simulink model "SimscapeCrane_StepInput"  (R2015a)
settings: Solver=ode15s  StartTime=0.0  StopTime=T  RelTol=1e-3
values from neighbouring files (symbols this model uses):
  filter_denominator = cell2mat(disc_filter.den)    [test.m]
  filter_numerator = cell2mat(disc_filter.num)    [test.m]
  m = 0.47    [Params_Simscape.mat]
  MR = 1.71    [Params_Simscape.mat]
  Ts_hw = 0.01    [test.m]
  TxBreak = 0    [Params_Simscape.mat]
  TxCoulomb = 3.7489    [Params_Simscape.mat]
  TxVisc = 58.085    [Params_Simscape.mat]
  TyBreak = 0    [Params_Simscape.mat]
  TyCoulomb = 2.674    [Params_Simscape.mat]
  TzBreak = 0    [Params_Simscape.mat]
  TzCoulomb = 6.1    [Params_Simscape.mat]
  xRange = [0 0.52]    [Params_Simscape.mat]
  xZero = 0.3    [Params_Simscape.mat]
  yRange = [0 0.62]    [Params_Simscape.mat]
  yZero = 0.3    [Params_Simscape.mat]
  zRange = [0.17 0.8]    [Params_Simscape.mat]
  zZero = 0.47    [Params_Simscape.mat]
undefined symbols (not defined in the file or in its folder): Ts, X, x_init, Y, Z
undefined symbols (not defined in the file): M, TorqueMultX, TorqueMultY, TorqueMultZ, TxTrans, TyTrans, TyVisc, TzTrans, TzVisc
libraries: sm_lib x146, fl_lib x62, nesl_utility x24, elec_lib x9, simulink x9, sm_double_wishbone_suspension_lib x4, aerolibtransform2 x1
(part 1 of 15)
settings Model: Creator=jsustare  LastModifiedBy=bkhusain
settings SolverCC: MaxConsecutiveMinStep=10  AutoInsertRateTranBlk=on  InsertRTBMode=Never (minimum delay)
settings DataIOCC: LimitDataPoints=off  SaveFormat=StructureWithTime
settings HardwareCC: ProdBitPerPointer=64  ProdLargestAtomicFloat=Float  ProdIntDivRoundTo=Zero  ProdEndianess=LittleEndian  ProdHWDeviceType=Specified
settings SFSimCC: SimUserIncludeDirs=../../src
settings SFSimCC: SimUserSources=|
  | user_block.c
  | user_bounds.c
  | user_gradient.c
  | user_hessians.c
  | user_jacobians.c
  | user_residual.c
  | user_mv_mult_prescaled.c
  | user_prescaler.c
  | user_rec_sol.c
  | user_minres.c
  | user_lanczos.c
  | user_nlp_solver.c
  | soc_simulink_wrapper.c
settings GRTTargetCC: GeneratePreprocessorConditionals=Use local settings

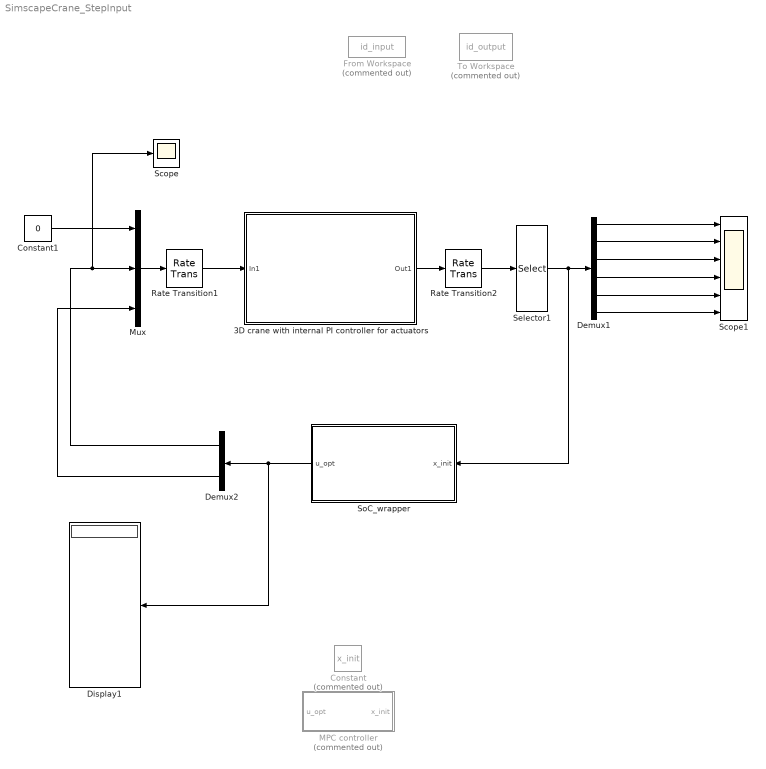
== system SimscapeCrane_StepInput ==
  3D crane with internal PI controller for actuators : Subsystem
  Constant : Constant  Commented=on  Value=x_init  SampleTime=Ts
  Constant1 : Constant  Value=0
  Demux1 : Demux  Outputs=6
  Demux2 : Demux  Outputs=2
  Display1 : Display
  From Workspace : FromWorkspace  Commented=on  VariableName=id_input  SampleTime=Ts
  MPC controller : Subsystem  Commented=on
  Mux : Mux  Inputs=3
  Rate Transition1 : RateTransition  Integrity=off  Deterministic=off  OutPortSampleTime=Ts_hw
  Rate Transition2 : RateTransition  Integrity=off  Deterministic=off  OutPortSampleTime=Ts
  Scope : Scope
      settings: SaveName=ScopeData4
  Scope1 : Scope  NumInputPorts=6
      settings: YMin=0.199~-0.035~0.49825~0~-0.015~-0.03  YMax=0.2035~0.015~0.50025~0.0035~0.01~0.04  SaveName=ScopeData5
  Selector1 : Selector  InputPortWidth=10  Indices=[3 4 5 6 9 10]
  SoC_wrapper : MATLAB Function  TreatAsAtomicUnit=on
  To Workspace : ToWorkspace  Commented=on  VariableName=id_output  SaveFormat=Structure With Time  SampleTime=Ts
  wires:
  3D crane with internal PI controller for actuators/1(Out1) -> Rate Transition2/1
  Mux/1 -> Rate Transition1/1
  Constant1/1 -> Mux/1
  Selector1/1 -> SoC_wrapper/1(x_init), Demux1/1
  Rate Transition1/1 -> 3D crane with internal PI controller for actuators/1(In1)
  Rate Transition2/1 -> Selector1/1
  Demux1/2 -> Scope1/2
  Demux1/4 -> Scope1/4
  Demux1/3 -> Scope1/3
  Demux1/1 -> Scope1/1
  Demux1/6 -> Scope1/6
  Demux1/5 -> Scope1/5
  Demux2/1 -> Scope/1, Mux/2
  Demux2/2 -> Mux/3
  SoC_wrapper/1(u_opt) -> Demux2/1, Display1/1
